simulink model "Simulation_of_Wind_Turbine_for_Household_Applications"  (R2018a)
settings: Solver=ode23tb  StartTime=0.0  StopTime=1  RelTol=1e-3
libraries: powerlib x45, powerlib_meascontrol x7, simulink x4
settings Model: Creator=engrf  LastModifiedBy=SAAD MAZHAR
settings SFSimCC: SimUseLocalCustomCode=on
settings RTWCC: RTWUseLocalCustomCode=on

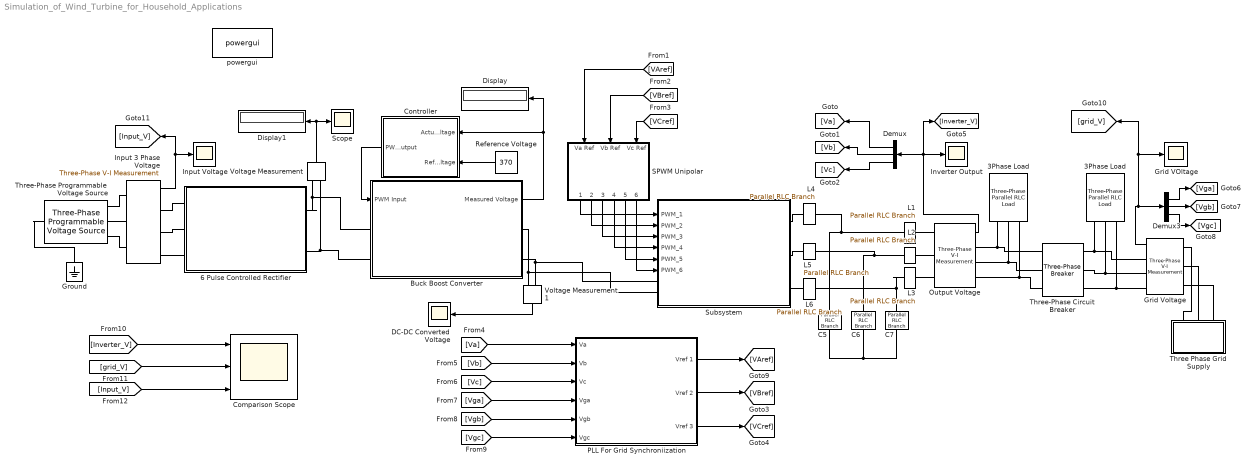
== system Simulation_of_Wind_Turbine_for_Household_Applications ==
  " Grid VOltage " : Scope
  "3Phase Load " : powerlib/Elements/Three-Phase Parallel RLC Load  LConnTagsString=A|B|C  Configuration=Y (grounded)  NominalVoltage=376  Vabc=[1e3 1e3 1e3]  Vabcp=[1e3 1e3 1e3]  NominalFrequency=50  UnbalancedPower=off  ActivePower=1000  InductivePower=0  CapacitivePower=0  Pabc=[10e3 9e3 11e3]  QLabc=[100 90 110]  QCabc=[100 90 110]  Pabcp=[10e3 9e3 11e3]  QLabcp=[100 90 110]  QCabcp=[100 90 110]  Measurements=None  LoadType=constant Z
      settings: SourceProductName=Simscape Electrical
  "3Phase Load " : powerlib/Elements/Three-Phase Parallel RLC Load  LConnTagsString=A|B|C  Configuration=Y (grounded)  NominalVoltage=376  Vabc=[1e3 1e3 1e3]  Vabcp=[1e3 1e3 1e3]  NominalFrequency=50  UnbalancedPower=off  ActivePower=1000  InductivePower=0  CapacitivePower=0  Pabc=[10e3 9e3 11e3]  QLabc=[100 90 110]  QCabc=[100 90 110]  Pabcp=[10e3 9e3 11e3]  QLabcp=[100 90 110]  QCabcp=[100 90 110]  Measurements=None  LoadType=constant Z
      settings: SourceProductName=Simscape Electrical
  6 Pulse Controlled Rectifier : Subsystem
  Buck Boost Converter : Subsystem
  C5 : powerlib/Elements/Parallel RLC Branch  LConnTagsString=a  RConnTagsString=__new0  BranchType=C  Resistance=inf  Inductance=inf  SetiL0=off  InitialCurrent=0  Capacitance=33.77e-6  Setx0=off  InitialVoltage=0  Measurements=None
      settings: SourceProductName=Simscape Electrical
  C6 : powerlib/Elements/Parallel RLC Branch  LConnTagsString=a  RConnTagsString=__new0  BranchType=C  Resistance=inf  Inductance=inf  SetiL0=off  InitialCurrent=0  Capacitance=33.77e-6  Setx0=off  InitialVoltage=0  Measurements=None
      settings: SourceProductName=Simscape Electrical
  C7 : powerlib/Elements/Parallel RLC Branch  LConnTagsString=a  RConnTagsString=__new0  BranchType=C  Resistance=inf  Inductance=inf  SetiL0=off  InitialCurrent=0  Capacitance=33.77e-6  Setx0=off  InitialVoltage=0  Measurements=None
      settings: SourceProductName=Simscape Electrical
  Comparison Scope : Scope  NumInputPorts=3
  "Controller " : Subsystem
  DC-DC Converted Voltage : Scope
  Demux : Demux  Outputs=3
  Demux3 : Demux  Outputs=3
  Display : Display
  Display1 : Display
  Grid Voltage : powerlib/Measurements/Three-Phase V-I Measurement  VoltageMeasurement=phase-to-ground  SetLabelV=off  LabelV=grid_V  Vpu=off  VpuLL=off  CurrentMeasurement=no  SetLabelI=off  LabelI=Iabc  Ipu=off  Pbase=100e6  Vbase=500e3  OutputType=Complex  PhasorSimulation=off  PSBequivalent=0
      settings: SourceProductName=Simscape Electrical
  Ground : powerlib/Elements/Ground  LConnTagsString=a
      settings: SourceProductName=Simscape Electrical
  Input 3 Phase Voltage : powerlib/Measurements/Three-Phase V-I Measurement  VoltageMeasurement=phase-to-ground  SetLabelV=off  LabelV=Vabc  Vpu=off  VpuLL=off  CurrentMeasurement=no  SetLabelI=off  LabelI=Iabc  Ipu=off  Pbase=100e6  Vbase=500e3  OutputType=Complex  PhasorSimulation=off  PSBequivalent=0
      settings: SourceProductName=Simscape Electrical
  Input Voltage : Scope
  "Inverter Output " : Scope
  L{1..6} (6 alike) : powerlib/Elements/Parallel RLC Branch  LConnTagsString=a  RConnTagsString=__new0  BranchType=L  Resistance=inf  Inductance=300e-3  SetiL0=off  InitialCurrent=0  Capacitance=1.3e-3  Setx0=off  InitialVoltage=0  Measurements=None
      settings: SourceProductName=Simscape Electrical
  Output Voltage : powerlib/Measurements/Three-Phase V-I Measurement  VoltageMeasurement=phase-to-ground  SetLabelV=off  LabelV=Inverter_V  Vpu=off  VpuLL=off  CurrentMeasurement=no  SetLabelI=off  LabelI=Iabc  Ipu=off  Pbase=100e6  Vbase=500e3  OutputType=Complex  PhasorSimulation=off  PSBequivalent=0
      settings: SourceProductName=Simscape Electrical
  PLL For Grid Synchroniization : Subsystem
  Reference Voltage : Constant  Value=370
  SPWM Unipolar : Subsystem
  Scope : Scope
  Subsystem : Subsystem
  Three Phase Grid Supply : Subsystem
  Three-Phase Programmable Voltage Source : powerlib/Electrical Sources/Three-Phase Programmable Voltage Source  PositiveSequence="[440  0 50]"  VariationEntity=Amplitude  VariationType=Table of time-amplitude pairs  VariationTypeAlt=Step  VariationStep=10  VariationRate=10  VariationMagnitude=0.3  VariationFrequency=2  VariationTiming=[0.5 1]  VariationPhaseA=off  Amplitudes=[1 0.77 0.6 1.0]  TimeValues=[0 0.25 0.5 0.75]  HarmonicGeneration=off  HarmonicA=[3 0.2 -25 0]  HarmonicB=[2 0.15 35 2]  Timing="[0.05  3]"  BusType=swing  Pref=0  Qref=0  Qmin=-inf  Qmax=inf
      settings: SourceProductName=Simscape Electrical
  Three-Phase Circuit Breaker : powerlib/Elements/Three-Phase Breaker  InitialState=open  SwitchA=on  SwitchB=on  SwitchC=on  SwitchTimes=[0 100]  External=off  BreakerResistance=0.01  SnubberResistance=1e6  SnubberCapacitance=inf  Measurements=None
      settings: SourceProductName=Simscape Electrical
  Voltage Measurement : powerlib/Measurements/Voltage Measurement  PhasorSimulation=off  OutputType=Complex  PSBequivalent=0
      settings: SourceProductName=Simscape Electrical
  Voltage Measurement1 : powerlib/Measurements/Voltage Measurement  PhasorSimulation=off  OutputType=Complex  PSBequivalent=0
      settings: SourceProductName=Simscape Electrical
  powergui : powerlib/powergui  Priority=1  SimulationMode=Continuous  SampleTime=50e-6  frequency=60  Iterations=50  frequencyindice=0  Pbase=100e6  ErrMax=1e-4  UnitsV=kV  UnitsW=MW  buscounter=0  FunctionMessages=off  echomessages=off  EnableUseOfTLC=off  CurrentSourceSwitches=off  DisableSnubberDevices=off  DisableRonSwitches=off  DisableVfSwitches=off  DisplayEquations=off  SolverType=Tustin/Backward Euler (TBE)  Interpol=off  ExternalGateDelay=off  methode=off  Ts=100  x0status=blocks  SPID=on  SwTol=0  HookPort=off  RestoreLinks=warning  ResistiveCurrentMeasurement=off  Frange=[0:2:500]  Ylog=off  Xlog=on  ShowGrid=off  save=off  variable=ZData  structure=BuckBoost_Voltage  ZoomFFT=off  StartTime=0.35  cycles=10  DisplayStyle=5  fundamental=50  FreqAxis=on  MaxFrequency=500  frequencyindicesteady=1  RmsSteady=1  display=off
  wires:
  Voltage Measurement/1 -> Scope/1, Display1/1
  Input 3 Phase Voltage/1 -> [Input_V], Input Voltage/1
  Buck Boost Converter/1(Measured Voltage) -> Display/1, "Controller "/1(Actual Voltage)
  Reference Voltage/1 -> "Controller "/2(Reference Voltage)
  Voltage Measurement1/1 -> DC-DC Converted Voltage/1
  "Controller "/1(PWM output) -> Buck Boost Converter/1(PWM Input)
  Demux/1 -> [Va]
  [VBref] -> SPWM Unipolar/2(Vb Ref)
  [Vb] -> PLL For Grid Synchroniization/2(Vb)
  [VCref] -> SPWM Unipolar/3(Vc Ref)
  [VAref] -> SPWM Unipolar/1(Va Ref)
  PLL For Grid Synchroniization/2(Vref 2) -> [VBref]
  [Inverter_V] -> Comparison Scope/1
  [Vc] -> PLL For Grid Synchroniization/3(Vc)
  Output Voltage/1 -> [Inverter_V], Demux/1, "Inverter Output "/1
  [grid_V] -> Comparison Scope/2
  [Vga] -> PLL For Grid Synchroniization/4(Vga)
  Demux3/1 -> [Vga]
  Grid Voltage/1 -> " Grid VOltage "/1, [grid_V], Demux3/1
  SPWM Unipolar/1(PWM 1) -> Subsystem/1(PWM_1)
  SPWM Unipolar/6("PWM 6 ") -> Subsystem/6(PWM_6)
  SPWM Unipolar/3(PWM 3) -> Subsystem/3(PWM_3)
  SPWM Unipolar/2(PWM 2) -> Subsystem/2(PWM_2)
  SPWM Unipolar/4(PWM 4) -> Subsystem/4(PWM_4)
  [Vgc] -> PLL For Grid Synchroniization/6(Vgc)
  Demux3/3 -> [Vgc]
  SPWM Unipolar/5(PWM 5) -> Subsystem/5(PWM_5)
  PLL For Grid Synchroniization/3(Vref 3) -> [VCref]
  PLL For Grid Synchroniization/1(Vref 1) -> [VAref]
  [Va] -> PLL For Grid Synchroniization/1("Va ")
  [Vgb] -> PLL For Grid Synchroniization/5(Vgb)
  Demux/3 -> [Vc]
  Demux3/2 -> [Vgb]
  Demux/2 -> [Vb]
  [Input_V] -> Comparison Scope/3
  connections:
  6 Pulse Controlled Rectifier/RConn2 -- Buck Boost Converter/LConn2 -- Voltage Measurement/LConn2
  Three-Phase Programmable Voltage Source/RConn3 -- Input 3 Phase Voltage/LConn3
  6 Pulse Controlled Rectifier/LConn1 -- Input 3 Phase Voltage/RConn1
  Three-Phase Programmable Voltage Source/RConn1 -- Input 3 Phase Voltage/LConn1
  Three-Phase Programmable Voltage Source/RConn2 -- Input 3 Phase Voltage/LConn2
  Three-Phase Programmable Voltage Source/LConn1 -- Ground/LConn1
  6 Pulse Controlled Rectifier/LConn2 -- Input 3 Phase Voltage/RConn2
  6 Pulse Controlled Rectifier/RConn1 -- Buck Boost Converter/LConn1 -- Voltage Measurement/LConn1
  6 Pulse Controlled Rectifier/LConn3 -- Input 3 Phase Voltage/RConn3
  Voltage Measurement1/LConn2 -- Subsystem/LConn2 -- Buck Boost Converter/RConn1
  Voltage Measurement1/LConn1 -- Subsystem/LConn1 -- Buck Boost Converter/RConn2
  Three-Phase Circuit Breaker/LConn2 -- "3Phase Load "/LConn2 -- Output Voltage/RConn2
  Grid Voltage/RConn1 -- Three-Phase Circuit Breaker/RConn1 -- "3Phase Load "/LConn1
  Three-Phase Circuit Breaker/LConn1 -- "3Phase Load "/LConn1 -- Output Voltage/RConn1
  C6/LConn1 -- L2/LConn1 -- L5/RConn1
  "3Phase Load "/LConn2 -- Three-Phase Circuit Breaker/RConn2 -- Grid Voltage/RConn2
  C5/RConn1 -- C6/RConn1 -- C7/RConn1
  L3/LConn1 -- L6/RConn1 -- C7/LConn1
  Three-Phase Circuit Breaker/RConn3 -- "3Phase Load "/LConn3 -- Grid Voltage/RConn3
  C5/LConn1 -- L1/LConn1 -- L4/RConn1
  Output Voltage/RConn3 -- Three-Phase Circuit Breaker/LConn3 -- "3Phase Load "/LConn3
  Three Phase Grid Supply/RConn3 -- Grid Voltage/LConn3
  L6/LConn1 -- Subsystem/RConn3
  L5/LConn1 -- Subsystem/RConn2
  L1/RConn1 -- Output Voltage/LConn1
  Three Phase Grid Supply/RConn2 -- Grid Voltage/LConn2
  L4/LConn1 -- Subsystem/RConn1
  Three Phase Grid Supply/RConn1 -- Grid Voltage/LConn1
  L2/RConn1 -- Output Voltage/LConn2
  L3/RConn1 -- Output Voltage/LConn3

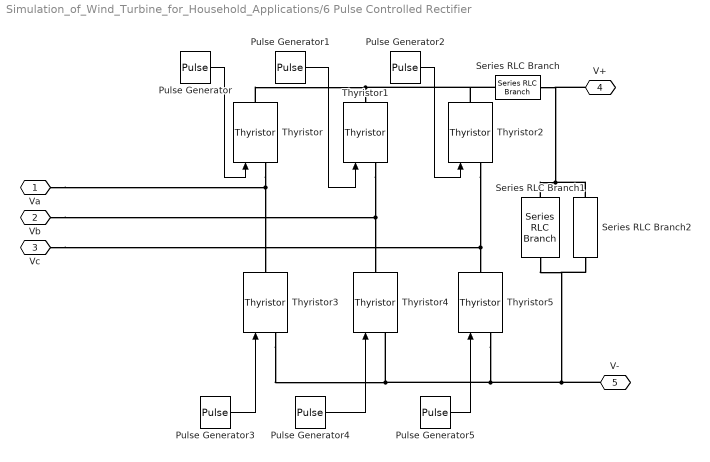
== system Simulation_of_Wind_Turbine_for_Household_Applications/6 Pulse Controlled Rectifier ==
  Pulse Generator : DiscretePulseGenerator  PulseType=Time based  Amplitude=10  Period=0.02  PulseWidth=50  PhaseDelay=(50)*(0.02)/360
  Pulse Generator1 : DiscretePulseGenerator  PulseType=Time based  Amplitude=10  Period=0.02  PulseWidth=50  PhaseDelay=(50+120)*(0.02)/360
  Pulse Generator2 : DiscretePulseGenerator  PulseType=Time based  Amplitude=10  Period=0.02  PulseWidth=50  PhaseDelay=(50+240)*(0.02)/360
  Pulse Generator3 : DiscretePulseGenerator  PulseType=Time based  Amplitude=10  Period=0.02  PulseWidth=50  PhaseDelay=(50+180)*(0.02)/360
  Pulse Generator4 : DiscretePulseGenerator  PulseType=Time based  Amplitude=10  Period=0.02  PulseWidth=50  PhaseDelay=(50+300)*(0.02)/360
  Pulse Generator5 : DiscretePulseGenerator  PulseType=Time based  Amplitude=10  Period=0.02  PulseWidth=50  PhaseDelay=(50+60)*(0.02)/360
  Series RLC Branch : powerlib/Elements/Series RLC Branch  LConnTagsString=__new0  RConnTagsString=__new0  BranchType=L  Resistance=1  Inductance=45e-3  SetiL0=off  InitialCurrent=0  Capacitance=1e-6  Setx0=off  InitialVoltage=0  Measurements=None
      settings: SourceProductName=Simscape Electrical
  Series RLC Branch1 : powerlib/Elements/Series RLC Branch  LConnTagsString=__new0  RConnTagsString=__new0  BranchType=C  Resistance=1  Inductance=1e-3  SetiL0=off  InitialCurrent=0  Capacitance=225.07e-6  Setx0=off  InitialVoltage=0  Measurements=None
      settings: SourceProductName=Simscape Electrical
  Series RLC Branch2 : powerlib/Elements/Series RLC Branch  LConnTagsString=__new0  RConnTagsString=__new0  BranchType=R  Resistance=10  Inductance=0.01  SetiL0=off  InitialCurrent=0  Capacitance=1e-6  Setx0=off  InitialVoltage=0  Measurements=Branch voltage and current
      settings: SourceProductName=Simscape Electrical
  Thyristor{,1..5} (6 alike) : powerlib/Power Electronics/Thyristor  Ron=0.001  Lon=0  Vf=0.8  IC=0  Rs=500  Cs=250e-9  Measurements=off
      settings: SourceProductName=Simscape Electrical
  Va : PMIOPort  Side=Left
  Vb : PMIOPort  Port=2  Side=Left
  Vc : PMIOPort  Port=3  Side=Left
  V+ : PMIOPort  Port=4  Side=Right
  V- : PMIOPort  Port=5  Side=Right
  wires:
  Pulse Generator/1 -> Thyristor/1
  Pulse Generator2/1 -> Thyristor2/1
  Pulse Generator1/1 -> Thyristor1/1
  Pulse Generator3/1 -> Thyristor3/1
  Pulse Generator4/1 -> Thyristor4/1
  Pulse Generator5/1 -> Thyristor5/1
  connections:
  Thyristor/RConn1 -- Series RLC Branch/LConn1 -- Thyristor2/RConn1 -- Thyristor1/RConn1
  Thyristor/LConn1 -- Va/RConn1 -- Thyristor3/RConn1
  Thyristor2/LConn1 -- Vc/RConn1 -- Thyristor5/RConn1
  Thyristor3/LConn1 -- Series RLC Branch2/RConn1 -- Series RLC Branch1/RConn1 -- V-/RConn1 -- Thyristor5/LConn1 -- Thyristor4/LConn1
  Thyristor1/LConn1 -- Vb/RConn1 -- Thyristor4/RConn1
  Series RLC Branch2/LConn1 -- V+/RConn1 -- Series RLC Branch/RConn1 -- Series RLC Branch1/LConn1

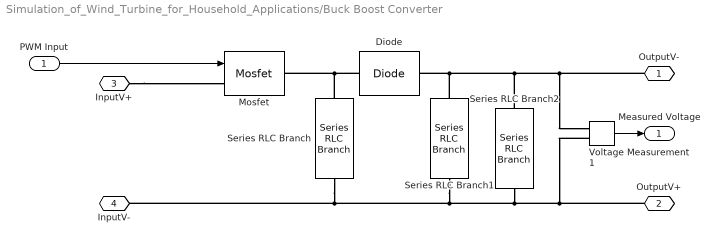
== system Simulation_of_Wind_Turbine_for_Household_Applications/Buck Boost Converter ==
  PWM Input : Inport
  Diode : powerlib/Power Electronics/Diode  Ron=0.001  Lon=0  Vf=0.8  IC=0  UseSnubber=0  Rs=500  Cs=250e-9  Measurements=off
      settings: SourceProductName=Simscape Electrical
  Mosfet : powerlib/Power Electronics/Mosfet  Ron=0.1  Lon=0  Rd=0.01  Vfd=0  IC=0  Rs=1e5  Cs=inf  Measurements=off
      settings: SourceProductName=Simscape Electrical
  Series RLC Branch : powerlib/Elements/Series RLC Branch  LConnTagsString=__new0  RConnTagsString=__new0  BranchType=L  Resistance=10  Inductance=10e-6  SetiL0=off  InitialCurrent=0  Capacitance=1e-6  Setx0=off  InitialVoltage=0  Measurements=None
      settings: SourceProductName=Simscape Electrical
  Series RLC Branch1 : powerlib/Elements/Series RLC Branch  LConnTagsString=__new0  RConnTagsString=__new0  BranchType=C  Resistance=10  Inductance=0.01  SetiL0=off  InitialCurrent=0  Capacitance=5e-3  Setx0=off  InitialVoltage=0  Measurements=None
      settings: SourceProductName=Simscape Electrical
  Series RLC Branch2 : powerlib/Elements/Series RLC Branch  LConnTagsString=__new0  RConnTagsString=__new0  BranchType=R  Resistance=100  Inductance=0.01  SetiL0=off  InitialCurrent=0  Capacitance=500  Setx0=off  InitialVoltage=0  Measurements=None
      settings: SourceProductName=Simscape Electrical
  Voltage Measurement1 : powerlib/Measurements/Voltage Measurement  PhasorSimulation=off  OutputType=Complex  PSBequivalent=0
      settings: SourceProductName=Simscape Electrical
  OutputV- : PMIOPort  Side=Right
  OutputV+ : PMIOPort  Port=2  Side=Right
  InputV+ : PMIOPort  Port=3  Side=Left
  InputV- : PMIOPort  Port=4  Side=Left
  Measured Voltage : Outport  VectorParamsAs1DForOutWhenUnconnected=on
  wires:
  PWM Input/1 -> Mosfet/1
  Voltage Measurement1/1 -> Measured Voltage/1
  connections:
  Series RLC Branch1/RConn1 -- Series RLC Branch/RConn1 -- InputV-/RConn1 -- OutputV+/RConn1 -- Voltage Measurement1/LConn2 -- Series RLC Branch2/RConn1
  Series RLC Branch1/LConn1 -- Diode/LConn1 -- OutputV-/RConn1 -- Voltage Measurement1/LConn1 -- Series RLC Branch2/LConn1
  Diode/RConn1 -- Series RLC Branch/LConn1 -- Mosfet/RConn1
  InputV+/RConn1 -- Mosfet/LConn1

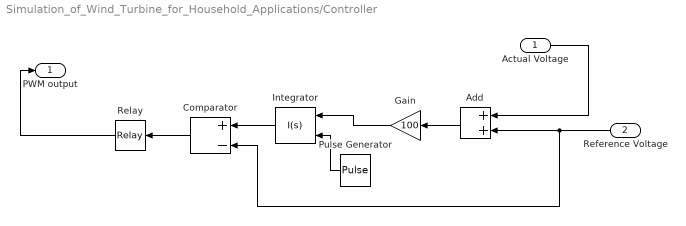
== system Simulation_of_Wind_Turbine_for_Household_Applications/Controller  ==
  Actual Voltage : Inport
  Reference Voltage : Inport  Port=2
  Add : Sum
  Comparator : Sum  Inputs=+-
  Gain : Gain  Gain=100
  Integrator : simulink/Continuous/PID Controller  Controller=I  TimeDomain=Continuous-time  SampleTime=-1  IntegratorMethod=Forward Euler  FilterMethod=Forward Euler  Form=Parallel  UseFilter=on  ControllerParametersSource=internal  P=1  I=40000  D=0  N=100  InitialConditionSource=internal  InitialConditionForIntegrator=0  InitialConditionForFilter=0  ExternalReset=rising  LimitOutput=off  UpperSaturationLimit=inf  LowerSaturationLimit=-inf  LinearizeAsGain=on  AntiWindupMode=none  Kb=1  TrackingMode=off  Kt=1  PParamMin=[]  PParamMax=[]  IParamMin=[]  IParamMax=[]  DParamMin=[]  DParamMax=[]  NParamMin=[]  NParamMax=[]  KbParamMin=[]  KbParamMax=[]  KtParamMin=[]  KtParamMax=[]  POutMin=[]  POutMax=[]  IOutMin=[]  IOutMax=[]  DOutMin=[]  DOutMax=[]  NOutMin=[]  NOutMax=[]  KbOutMin=[]  KbOutMax=[]  KtOutMin=[]  KtOutMax=[]  IntegratorOutMin=[]  IntegratorOutMax=[]  FilterOutMin=[]  FilterOutMax=[]  SumOutMin=[]  SumOutMax=[]  SumI1OutMin=[]  SumI1OutMax=[]  SumI2OutMin=[]  SumI2OutMax=[]  SumI3OutMin=[]  SumI3OutMax=[]  SumDOutMin=[]  SumDOutMax=[]  SaturationOutMin=[]  SaturationOutMax=[]  IntegratorContinuousStateAttributes=''  IntegratorStateMustResolveToSignalObject=off  IntegratorRTWStateStorageClass=Auto  FilterContinuousStateAttributes=''  FilterStateMustResolveToSignalObject=off  FilterRTWStateStorageClass=Auto  DifferentiatorICPrevScaledInput=0  DifferentiatorOutMin=[]  DifferentiatorOutMax=[]  FilterDiffOutCoefMin=[]  FilterDiffOutCoefMax=[]  SumDenOutMin=[]  SumDenOutMax=[]  SumNumOutMin=[]  SumNumOutMax=[]  ReciprocalOutMin=[]  ReciprocalOutMax=[]  DivideOutMin=[]  DivideOutMax=[]  TunerSelectOption=Transfer Function Based (PID Tuner App)
  Pulse Generator : DiscretePulseGenerator  PulseType=Time based  Period=1/10000  PulseWidth=50
  Relay : Relay
  PWM output : Outport  VectorParamsAs1DForOutWhenUnconnected=on
  wires:
  Gain/1 -> Integrator/1
  Reference Voltage/1 -> Comparator/2, Add/2
  Comparator/1 -> Relay/1
  Add/1 -> Gain/1
  Integrator/1 -> Comparator/1
  Relay/1 -> PWM output/1
  Pulse Generator/1 -> Integrator/2
  Actual Voltage/1 -> Add/1

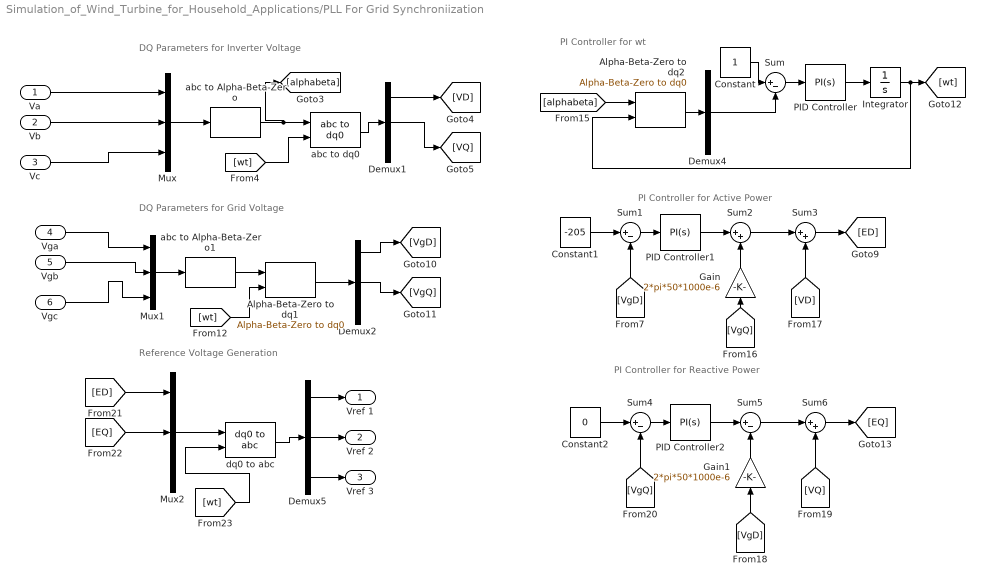
== system Simulation_of_Wind_Turbine_for_Household_Applications/PLL For Grid Synchroniization ==
  note: DQ Parameters for Inverter Voltage
  note: DQ Parameters for Grid Voltage
  note: Reference Voltage Generation
  note: PI Controller for Active Power
  note: PI Controller for Reactive Power
  note: PI Controller for wt
  "Va " : Inport
  Vb : Inport  Port=2
  Vc : Inport  Port=3
  Vga : Inport  Port=4
  Vgb : Inport  Port=5
  Vgc : Inport  Port=6
  Alpha-Beta-Zero to dq1 : powerlib_meascontrol/Transformations/Alpha-Beta-Zero to dq0  Alignment=90 degrees behind phase A axis
      settings: SourceProductName=Simscape Power Systems
  Alpha-Beta-Zero to dq2 : powerlib_meascontrol/Transformations/Alpha-Beta-Zero to dq0  Alignment=90 degrees behind phase A axis
      settings: SourceProductName=Simscape Power Systems
  Constant : Constant
  Constant1 : Constant  Value=-205
  Constant2 : Constant  Value=0
  Demux{1..2,4..5} (4 alike) : Demux  Outputs=3
  Gain : Gain  Gain=2*pi*50*1000e-6
  Gain1 : Gain  Gain=2*pi*50*1000e-6
  Integrator : Integrator
  Mux : Mux  Inputs=3
  Mux1 : Mux  Inputs=3
  Mux2 : Mux  Inputs=3
  PID Controller : simulink/Continuous/PID Controller  Controller=PI  TimeDomain=Continuous-time  SampleTime=-1  IntegratorMethod=Forward Euler  FilterMethod=Forward Euler  Form=Parallel  UseFilter=on  ControllerParametersSource=internal  P=10  I=50000  D=0  N=100  InitialConditionSource=internal  InitialConditionForIntegrator=0  InitialConditionForFilter=0  ExternalReset=none  LimitOutput=off  UpperSaturationLimit=inf  LowerSaturationLimit=-inf  LinearizeAsGain=on  AntiWindupMode=none  Kb=1  TrackingMode=off  Kt=1  PParamMin=[]  PParamMax=[]  IParamMin=[]  IParamMax=[]  DParamMin=[]  DParamMax=[]  NParamMin=[]  NParamMax=[]  KbParamMin=[]  KbParamMax=[]  KtParamMin=[]  KtParamMax=[]  POutMin=[]  POutMax=[]  IOutMin=[]  IOutMax=[]  DOutMin=[]  DOutMax=[]  NOutMin=[]  NOutMax=[]  KbOutMin=[]  KbOutMax=[]  KtOutMin=[]  KtOutMax=[]  IntegratorOutMin=[]  IntegratorOutMax=[]  FilterOutMin=[]  FilterOutMax=[]  SumOutMin=[]  SumOutMax=[]  SumI1OutMin=[]  SumI1OutMax=[]  SumI2OutMin=[]  SumI2OutMax=[]  SumI3OutMin=[]  SumI3OutMax=[]  SumDOutMin=[]  SumDOutMax=[]  SaturationOutMin=[]  SaturationOutMax=[]  IntegratorContinuousStateAttributes=''  IntegratorStateMustResolveToSignalObject=off  IntegratorRTWStateStorageClass=Auto  FilterContinuousStateAttributes=''  FilterStateMustResolveToSignalObject=off  FilterRTWStateStorageClass=Auto  DifferentiatorICPrevScaledInput=0  DifferentiatorOutMin=[]  DifferentiatorOutMax=[]  FilterDiffOutCoefMin=[]  FilterDiffOutCoefMax=[]  SumDenOutMin=[]  SumDenOutMax=[]  SumNumOutMin=[]  SumNumOutMax=[]  ReciprocalOutMin=[]  ReciprocalOutMax=[]  DivideOutMin=[]  DivideOutMax=[]  TunerSelectOption=Transfer Function Based (PID Tuner App)
  PID Controller1 : simulink/Continuous/PID Controller  Controller=PI  TimeDomain=Continuous-time  SampleTime=-1  IntegratorMethod=Forward Euler  FilterMethod=Forward Euler  Form=Parallel  UseFilter=on  ControllerParametersSource=internal  P=5  I=50000  D=0  N=100  InitialConditionSource=internal  InitialConditionForIntegrator=0  InitialConditionForFilter=0  ExternalReset=none  LimitOutput=off  UpperSaturationLimit=inf  LowerSaturationLimit=-inf  LinearizeAsGain=on  AntiWindupMode=none  Kb=1  TrackingMode=off  Kt=1  PParamMin=[]  PParamMax=[]  IParamMin=[]  IParamMax=[]  DParamMin=[]  DParamMax=[]  NParamMin=[]  NParamMax=[]  KbParamMin=[]  KbParamMax=[]  KtParamMin=[]  KtParamMax=[]  POutMin=[]  POutMax=[]  IOutMin=[]  IOutMax=[]  DOutMin=[]  DOutMax=[]  NOutMin=[]  NOutMax=[]  KbOutMin=[]  KbOutMax=[]  KtOutMin=[]  KtOutMax=[]  IntegratorOutMin=[]  IntegratorOutMax=[]  FilterOutMin=[]  FilterOutMax=[]  SumOutMin=[]  SumOutMax=[]  SumI1OutMin=[]  SumI1OutMax=[]  SumI2OutMin=[]  SumI2OutMax=[]  SumI3OutMin=[]  SumI3OutMax=[]  SumDOutMin=[]  SumDOutMax=[]  SaturationOutMin=[]  SaturationOutMax=[]  IntegratorContinuousStateAttributes=''  IntegratorStateMustResolveToSignalObject=off  IntegratorRTWStateStorageClass=Auto  FilterContinuousStateAttributes=''  FilterStateMustResolveToSignalObject=off  FilterRTWStateStorageClass=Auto  DifferentiatorICPrevScaledInput=0  DifferentiatorOutMin=[]  DifferentiatorOutMax=[]  FilterDiffOutCoefMin=[]  FilterDiffOutCoefMax=[]  SumDenOutMin=[]  SumDenOutMax=[]  SumNumOutMin=[]  SumNumOutMax=[]  ReciprocalOutMin=[]  ReciprocalOutMax=[]  DivideOutMin=[]  DivideOutMax=[]  TunerSelectOption=Transfer Function Based (PID Tuner App)
  PID Controller2 : simulink/Continuous/PID Controller  Controller=PI  TimeDomain=Continuous-time  SampleTime=-1  IntegratorMethod=Forward Euler  FilterMethod=Forward Euler  Form=Parallel  UseFilter=on  ControllerParametersSource=internal  P=5  I=50000  D=0  N=100  InitialConditionSource=internal  InitialConditionForIntegrator=0  InitialConditionForFilter=0  ExternalReset=none  LimitOutput=off  UpperSaturationLimit=inf  LowerSaturationLimit=-inf  LinearizeAsGain=on  AntiWindupMode=none  Kb=1  TrackingMode=off  Kt=1  PParamMin=[]  PParamMax=[]  IParamMin=[]  IParamMax=[]  DParamMin=[]  DParamMax=[]  NParamMin=[]  NParamMax=[]  KbParamMin=[]  KbParamMax=[]  KtParamMin=[]  KtParamMax=[]  POutMin=[]  POutMax=[]  IOutMin=[]  IOutMax=[]  DOutMin=[]  DOutMax=[]  NOutMin=[]  NOutMax=[]  KbOutMin=[]  KbOutMax=[]  KtOutMin=[]  KtOutMax=[]  IntegratorOutMin=[]  IntegratorOutMax=[]  FilterOutMin=[]  FilterOutMax=[]  SumOutMin=[]  SumOutMax=[]  SumI1OutMin=[]  SumI1OutMax=[]  SumI2OutMin=[]  SumI2OutMax=[]  SumI3OutMin=[]  SumI3OutMax=[]  SumDOutMin=[]  SumDOutMax=[]  SaturationOutMin=[]  SaturationOutMax=[]  IntegratorContinuousStateAttributes=''  IntegratorStateMustResolveToSignalObject=off  IntegratorRTWStateStorageClass=Auto  FilterContinuousStateAttributes=''  FilterStateMustResolveToSignalObject=off  FilterRTWStateStorageClass=Auto  DifferentiatorICPrevScaledInput=0  DifferentiatorOutMin=[]  DifferentiatorOutMax=[]  FilterDiffOutCoefMin=[]  FilterDiffOutCoefMax=[]  SumDenOutMin=[]  SumDenOutMax=[]  SumNumOutMin=[]  SumNumOutMax=[]  ReciprocalOutMin=[]  ReciprocalOutMax=[]  DivideOutMin=[]  DivideOutMax=[]  TunerSelectOption=Transfer Function Based (PID Tuner App)
  Sum{,1,4..5} (4 alike) : Sum  Inputs=|+-
  Sum2 : Sum  Inputs=|++
  Sum3 : Sum  Inputs=|++
  Sum6 : Sum  Inputs=|++
  abc to Alpha-Beta-Zero : powerlib_meascontrol/Transformations/abc to Alpha-Beta-Zero
      settings: SourceProductName=Simscape Power Systems
  abc to Alpha-Beta-Zero1 : powerlib_meascontrol/Transformations/abc to Alpha-Beta-Zero
      settings: SourceProductName=Simscape Power Systems
  abc to dq0 : powerlib_meascontrol/Transformations/abc to dq0  Alignment=90 degrees behind phase A axis
  dq0 to abc : powerlib_meascontrol/Transformations/dq0 to abc  Alignment=90 degrees behind phase A axis
  Vref 1 : Outport  VectorParamsAs1DForOutWhenUnconnected=on
  Vref 2 : Outport  Port=2  VectorParamsAs1DForOutWhenUnconnected=on
  Vref 3 : Outport  Port=3  VectorParamsAs1DForOutWhenUnconnected=on
  wires:
  Gain/1 -> Sum2/2
  [wt] -> Alpha-Beta-Zero to dq1/2
  Integrator/1 -> Alpha-Beta-Zero to dq2/2, [wt]
  [VgD] -> Sum1/2
  [alphabeta] -> Alpha-Beta-Zero to dq2/1
  Alpha-Beta-Zero to dq2/1 -> Demux4/1
  abc to Alpha-Beta-Zero/1 -> [alphabeta], abc to dq0/1
  Demux4/2 -> Sum/2
  PID Controller/1 -> Integrator/1
  [ED] -> Mux2/1
  Mux/1 -> abc to Alpha-Beta-Zero/1
  Vgb/1 -> Mux1/2
  Sum/1 -> PID Controller/1
  Demux2/2 -> [VgQ]
  Constant/1 -> Sum/1
  Constant2/1 -> Sum4/1
  [VD] -> Sum3/2
  abc to Alpha-Beta-Zero1/1 -> Alpha-Beta-Zero to dq1/1
  abc to dq0/1 -> Demux1/1
  Gain1/1 -> Sum5/2
  Sum6/1 -> [EQ]
  [wt] -> abc to dq0/2
  Alpha-Beta-Zero to dq1/1 -> Demux2/1
  [VQ] -> Sum6/2
  Demux2/1 -> [VgD]
  Demux1/1 -> [VD]
  Mux1/1 -> abc to Alpha-Beta-Zero1/1
  Sum1/1 -> PID Controller1/1
  [wt] -> dq0 to abc/2
  [EQ] -> Mux2/2
  Sum4/1 -> PID Controller2/1
  dq0 to abc/1 -> Demux5/1
  [VgQ] -> Sum4/2
  Sum3/1 -> [ED]
  Mux2/1 -> dq0 to abc/1
  Sum2/1 -> Sum3/1
  Constant1/1 -> Sum1/1
  PID Controller2/1 -> Sum5/1
  [VgQ] -> Gain/1
  [VgD] -> Gain1/1
  Demux1/2 -> [VQ]
  PID Controller1/1 -> Sum2/1
  Sum5/1 -> Sum6/1
  "Va "/1 -> Mux/1
  Vb/1 -> Mux/2
  Vc/1 -> Mux/3
  Vga/1 -> Mux1/1
  Vgc/1 -> Mux1/3
  Demux5/1 -> Vref 1/1
  Demux5/2 -> Vref 2/1
  Demux5/3 -> Vref 3/1

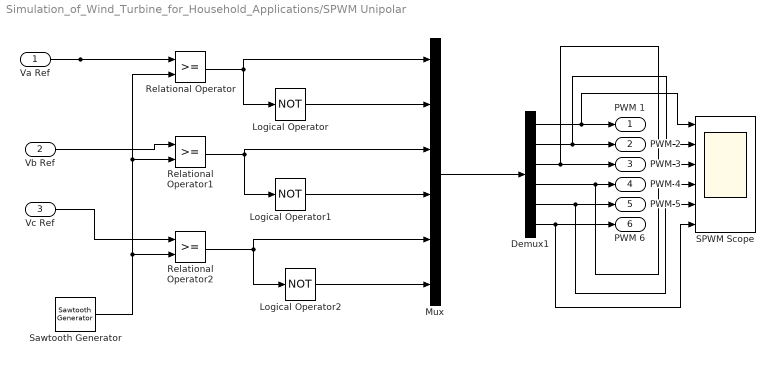
== system Simulation_of_Wind_Turbine_for_Household_Applications/SPWM Unipolar ==
  Va Ref : Inport
  Vb Ref : Inport  Port=2
  Vc Ref : Inport  Port=3
  Demux1 : Demux  Outputs=6
  Logical Operator : Logic  Operator=NOT  AllPortsSameDT=off  OutDataTypeStr=boolean
  Logical Operator1 : Logic  Operator=NOT  AllPortsSameDT=off  OutDataTypeStr=boolean
  Logical Operator2 : Logic  Operator=NOT  AllPortsSameDT=off  OutDataTypeStr=boolean
  Mux : Mux  Inputs=6
  Relational Operator : RelationalOperator  OutDataTypeStr=boolean  RndMeth=Nearest
  Relational Operator1 : RelationalOperator  OutDataTypeStr=boolean  RndMeth=Nearest
  Relational Operator2 : RelationalOperator  OutDataTypeStr=boolean  RndMeth=Nearest
  SPWM Scope : Scope  NumInputPorts=6
  Sawtooth Generator : powerlib_meascontrol/Pulse & Signal Generators/Sawtooth Generator  Freq=1e3  Phase=180  Ts=0
      settings: SourceProductName=Simscape Electrical
  PWM 1 : Outport  VectorParamsAs1DForOutWhenUnconnected=on
  PWM 2 : Outport  Port=2  VectorParamsAs1DForOutWhenUnconnected=on
  PWM 3 : Outport  Port=3  VectorParamsAs1DForOutWhenUnconnected=on
  PWM 4 : Outport  Port=4  VectorParamsAs1DForOutWhenUnconnected=on
  PWM 5 : Outport  Port=5  VectorParamsAs1DForOutWhenUnconnected=on
  "PWM 6 " : Outport  Port=6  VectorParamsAs1DForOutWhenUnconnected=on
  wires:
  Va Ref/1 -> Relational Operator/1
  Relational Operator1/1 -> Logical Operator1/1, Mux/3
  Sawtooth Generator/1 -> Relational Operator2/2, Relational Operator1/2, Relational Operator/2
  Logical Operator1/1 -> Mux/4
  Relational Operator/1 -> Logical Operator/1, Mux/1
  Logical Operator/1 -> Mux/2
  Mux/1 -> Demux1/1
  Relational Operator2/1 -> Logical Operator2/1, Mux/5
  Logical Operator2/1 -> Mux/6
  Vc Ref/1 -> Relational Operator2/1
  Vb Ref/1 -> Relational Operator1/1
  Demux1/1 -> SPWM Scope/1, PWM 1/1
  Demux1/5 -> SPWM Scope/5, PWM 5/1
  Demux1/2 -> SPWM Scope/2, PWM 2/1
  Demux1/4 -> SPWM Scope/4, PWM 4/1
  Demux1/6 -> SPWM Scope/6, "PWM 6 "/1
  Demux1/3 -> SPWM Scope/3, PWM 3/1

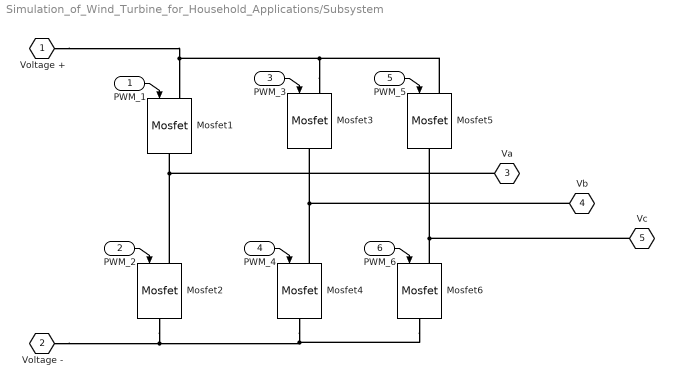
== system Simulation_of_Wind_Turbine_for_Household_Applications/Subsystem ==
  PWM_1 : Inport
  PWM_2 : Inport  Port=2
  PWM_3 : Inport  Port=3
  PWM_4 : Inport  Port=4
  PWM_5 : Inport  Port=5
  PWM_6 : Inport  Port=6
  Mosfet{1..6} (6 alike) : powerlib/Power Electronics/Mosfet  Ron=0.1  Lon=0  Rd=0.01  Vfd=0  IC=0  Rs=1e5  Cs=inf  Measurements=off
      settings: SourceProductName=Simscape Electrical
  Voltage + : PMIOPort  Side=Left
  Voltage - : PMIOPort  Port=2  Side=Left
  Va : PMIOPort  Port=3  Side=Right
  Vb : PMIOPort  Port=4  Side=Right
  Vc : PMIOPort  Port=5  Side=Right
  wires:
  PWM_2/1 -> Mosfet2/1
  PWM_5/1 -> Mosfet5/1
  PWM_1/1 -> Mosfet1/1
  PWM_4/1 -> Mosfet4/1
  PWM_6/1 -> Mosfet6/1
  PWM_3/1 -> Mosfet3/1
  connections:
  Mosfet4/LConn1 -- Vb/RConn1 -- Mosfet3/RConn1
  Mosfet3/LConn1 -- Mosfet5/LConn1 -- Voltage +/RConn1 -- Mosfet1/LConn1
  Mosfet6/LConn1 -- Mosfet5/RConn1 -- Vc/RConn1
  Mosfet2/LConn1 -- Va/RConn1 -- Mosfet1/RConn1
  Mosfet2/RConn1 -- Voltage -/RConn1 -- Mosfet4/RConn1 -- Mosfet6/RConn1

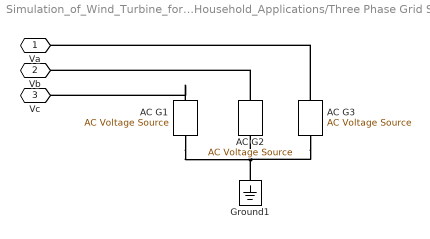
== system Simulation_of_Wind_Turbine_for_Household_Applications/Three Phase Grid Supply ==
  AC G1 : powerlib/Electrical Sources/AC Voltage Source  Amplitude=240  Phase=0  Frequency=50  SampleTime=0  Measurements=None  BusType=swing  Pref=10e3  Qref=0  Qmin=-inf  Qmax=+inf
      settings: SourceProductName=Simscape Electrical
  AC G2 : powerlib/Electrical Sources/AC Voltage Source  Amplitude=240  Phase=-120  Frequency=50  SampleTime=0  Measurements=None  BusType=swing  Pref=10e3  Qref=0  Qmin=-inf  Qmax=+inf
      settings: SourceProductName=Simscape Electrical
  AC G3 : powerlib/Electrical Sources/AC Voltage Source  Amplitude=240  Phase=120  Frequency=50  SampleTime=0  Measurements=None  BusType=swing  Pref=10e3  Qref=0  Qmin=-inf  Qmax=+inf
      settings: SourceProductName=Simscape Electrical
  Ground1 : powerlib/Elements/Ground  LConnTagsString=a
      settings: SourceProductName=Simscape Electrical
  Va : PMIOPort  Side=Right
  Vb : PMIOPort  Port=2  Side=Right
  Vc : PMIOPort  Port=3  Side=Right
  connections:
  AC G3/LConn1 -- AC G2/LConn1 -- Ground1/LConn1 -- AC G1/LConn1
  AC G1/RConn1 -- Vc/RConn1
  AC G2/RConn1 -- Vb/RConn1
  AC G3/RConn1 -- Va/RConn1
